simulink model "sampleModel20"  (R2021a)
settings: Solver=VariableStepAuto  StartTime=0.0  StopTime=10.0  RelTol=1e-3
undefined symbols (not defined in the file): DiscIntNeverNeededParam, magnitude, Newton, Raphson
libraries: simulink x274, pid_lib x17
(part 12 of 16)

== system sampleModel20/cfblk86/cfblk9/cfblk4/cfblk10 ==
  cfblk1 : Inport
  cfblk9 : Inport  Port=2
  cfblk10 : Inport  Port=3
  cfblk3 : Sqrt  Operator=rSqrt  AlgorithmType=Newton-Raphson  SaturateOnIntegerOverflow=on
  cfblk4 : UnaryMinus
  cfblk5 : Product  Inputs=*
  cfblk6 : PermuteDimensions
  cfblk7 : Sqrt  Operator=rSqrt  AlgorithmType=Newton-Raphson  SaturateOnIntegerOverflow=on
  cfblk8 : Sum  Inputs=+-
  cfblk2 : Outport
  wires:
  cfblk8/1 -> cfblk4/1
  cfblk6/1 -> cfblk2/1
  cfblk5/1 -> cfblk8/1
  cfblk1/1 -> cfblk7/1
  cfblk3/1 -> cfblk5/1
  cfblk10/1 -> cfblk8/2
  cfblk9/1 -> cfblk3/1
  cfblk4/1 -> cfblk6/1

== system sampleModel20/cfblk86/cfblk9/cfblk4/cfblk11 ==
  cfblk1 : Inport
  cfblk6 : Inport  Port=2
  cfblk7 : Inport  Port=3
  cfblk8 : Inport  Port=4
  cfblk9 : Inport  Port=5
  cfblk10 : Inport  Port=6
  cfblk3 : Squeeze
  cfblk4 : ComplexToMagnitudeAngle
  cfblk5 : Product  Inputs=*
  cfblk2 : Outport
  cfblk11 : Outport  Port=2
  wires:
  cfblk8/1 -> cfblk2/1
  cfblk6/1 -> cfblk4/1
  cfblk1/1 -> cfblk11/1
  cfblk4/1 -> cfblk5/1
  cfblk9/1 -> cfblk3/1

== system sampleModel20/cfblk86/cfblk9/cfblk4/cfblk12 ==
  cfblk1 : Inport
  cfblk9 : Inport  Port=2
  cfblk10 : Inport  Port=3
  cfblk11 : Inport  Port=4
  cfblk3 : Reshape
  cfblk4 : Math  Operator=mod  SaturateOnIntegerOverflow=on
  cfblk5 : DotProduct  InputSameDT=on  OutDataTypeStr=Inherit: Inherit via internal rule
  cfblk6 : Sum  Inputs=|++
  cfblk7 : Product  Inputs=**
  cfblk8 : PermuteDimensions
  cfblk2 : Outport
  wires:
  cfblk8/1 -> cfblk3/1
  cfblk11/1 -> cfblk7/1
  cfblk1/1 -> cfblk5/1
  cfblk3/1 -> cfblk7/2
  cfblk9/1 -> cfblk4/1
  cfblk10/1 -> cfblk4/2, cfblk5/2
  cfblk7/1 -> cfblk2/1
  cfblk6/1 -> cfblk8/1
  cfblk4/1 -> cfblk6/1
  cfblk5/1 -> cfblk6/2

== system sampleModel20/cfblk86/cfblk9/cfblk4/cfblk9 ==
  cfblk1 : Inport
  cfblk9 : Inport  Port=2
  cfblk10 : Inport  Port=3
  cfblk11 : Inport  Port=4
  cfblk13 : Delay  SampleTime=1
  cfblk3 : Squeeze
  cfblk4 : Sin  TimeSource=Use external signal  SampleTime=0
  cfblk5 : Sum  Inputs=+
  cfblk6 : simulink/Math Operations/MinMax Running Resettable  Function=min  vinit=0.0
  cfblk7 : Sum  Inputs=--
  cfblk8 : simulink/Math Operations/MinMax Running Resettable  Function=min  vinit=0.0
  cfblk2 : Outport
  cfblk12 : Outport  Port=2
  wires:
  cfblk8/1 -> cfblk4/1
  cfblk1/1 -> cfblk7/2
  cfblk10/1 -> cfblk2/1
  cfblk9/1 -> cfblk8/1
  cfblk7/1 -> cfblk3/1
  cfblk3/1 -> cfblk5/1, cfblk6/2
  cfblk11/1 -> cfblk8/2
  cfblk5/1 -> cfblk12/1
  cfblk4/1 -> cfblk6/1
  cfblk6/1 -> cfblk13/1
  cfblk13/1 -> cfblk7/1

== system sampleModel20/cfblk86/cfblk9/cfblk5/cfblk11 ==
  cfblk1 : Inport
  cfblk6 : Inport  Port=2
  cfblk7 : Inport  Port=3
  cfblk8 : Inport  Port=4
  cfblk9 : Inport  Port=5
  cfblk10 : Inport  Port=6
  cfblk11 : Inport  Port=7
  cfblk12 : Inport  Port=8
  cfblk3 : ComplexToMagnitudeAngle
  cfblk4 : Gain  Gain=[-542068454.447755]
  cfblk5 : Sqrt  SaturateOnIntegerOverflow=on
  cfblk2 : Outport
  cfblk13 : Outport  Port=2
  cfblk14 : Outport  Port=3
  cfblk15 : Outport  Port=4
  wires:
  cfblk3/1 -> cfblk5/1
  cfblk5/1 -> cfblk2/1
  cfblk7/1 -> cfblk4/1
  cfblk6/1 -> cfblk15/1
  cfblk10/1 -> cfblk3/1
  cfblk12/1 -> cfblk13/1
  cfblk3/2 -> cfblk14/1

== system sampleModel20/cfblk86/cfblk9/cfblk5/cfblk12 ==
  cfblk1 : Inport
  cfblk5 : Inport  Port=2
  cfblk6 : Inport  Port=3
  cfblk7 : Inport  Port=4
  cfblk3 : Assignment  DiagnosticForDimensions=Warning  IndexOptions=Index vector (dialog)  Indices=1  OutputSizes=1
  cfblk4 : Assignment  DiagnosticForDimensions=Warning  IndexOptions=Index vector (dialog)  Indices=1  OutputSizes=1
  cfblk2 : Outport
  cfblk8 : Outport  Port=2
  wires:
  cfblk6/1 -> cfblk4/1
  cfblk1/1 -> cfblk8/1
  cfblk7/1 -> cfblk3/1
  cfblk5/1 -> cfblk3/2
  cfblk4/1 -> cfblk2/1
  cfblk3/1 -> cfblk4/2

== system sampleModel20/cfblk86/cfblk9/cfblk6/cfblk6 ==
  cfblk1 : Inport
  cfblk8 : Inport  Port=2
  cfblk9 : Inport  Port=3
  cfblk10 : Inport  Port=4
  cfblk11 : Inport  Port=5
  cfblk3 : ComplexToRealImag
  cfblk4 : Polyval  Coefs=[ +2.081618890e-019, -1.441693666e-014, +4.719686976e-010, -8.536869453e-006, +1.621573104e-001, -8.087801117e+001 ]
  cfblk5 : ComplexToRealImag
  cfblk6 : Product  Inputs=**
  cfblk7 : Signum
  cfblk2 : Outport
  wires:
  cfblk11/1 -> cfblk6/1
  cfblk9/1 -> cfblk4/1
  cfblk10/1 -> cfblk7/1
  cfblk4/1 -> cfblk6/2
  cfblk3/1 -> cfblk5/1
  cfblk7/1 -> cfblk2/1
  cfblk1/1 -> cfblk3/1

== system sampleModel20/cfblk86/cfblk9/cfblk6/cfblk7 ==
  cfblk1 : Inport
  cfblk11 : Inport  Port=2
  cfblk12 : Inport  Port=3
  cfblk13 : Inport  Port=4
  cfblk14 : Inport  Port=5
  cfblk15 : Inport  Port=6
  cfblk10 : MinMax  Inputs=3
  cfblk3 : DiscreteFir  SampleTime=1
  cfblk4 : Assignment  DiagnosticForDimensions=Warning  IndexOptions=Index vector (dialog)  Indices=1  OutputSizes=1
  cfblk5 : Product  Inputs=**
  cfblk6 : Squeeze
  cfblk7 : Signum
  cfblk8 : ComplexToRealImag
  cfblk9 : Sqrt  Operator=rSqrt  AlgorithmType=Newton-Raphson  SaturateOnIntegerOverflow=on
  cfblk2 : Outport
  cfblk16 : Outport  Port=2
  wires:
  cfblk10/1 -> cfblk2/1
  cfblk13/1 -> cfblk6/1
  cfblk3/1 -> cfblk9/1
  cfblk12/1 -> cfblk7/1
  cfblk6/1 -> cfblk3/1
  cfblk4/1 -> cfblk16/1
  cfblk8/1 -> cfblk5/1
  cfblk7/1 -> cfblk8/1
  cfblk8/2 -> cfblk5/2
  cfblk9/1 -> cfblk10/1
  cfblk15/1 -> cfblk10/2
  cfblk1/1 -> cfblk10/3
  cfblk14/1 -> cfblk4/1
  cfblk5/1 -> cfblk4/2

== system sampleModel20/cfblk86/cfblk9/cfblk6/cfblk8 ==
  cfblk1 : Inport
  cfblk7 : Inport  Port=2
  cfblk8 : Inport  Port=3
  cfblk9 : Inport  Port=4
  cfblk10 : Inport  Port=5
  cfblk11 : Inport  Port=6
  cfblk3 : Sin  TimeSource=Use external signal  SampleTime=0
  cfblk4 : Product  Inputs=*
  cfblk5 : simulink/Math Operations/Slider Gain  gain=1  low=0  high=2
  cfblk6 : Reshape
  cfblk2 : Outport
  cfblk12 : Outport  Port=2
  cfblk13 : Outport  Port=3
  wires:
  cfblk1/1 -> cfblk6/1
  cfblk10/1 -> cfblk2/1
  cfblk8/1 -> cfblk12/1
  cfblk11/1 -> cfblk4/1
  cfblk7/1 -> cfblk3/1
  cfblk5/1 -> cfblk13/1
  cfblk3/1 -> cfblk5/1

== system sampleModel20/cfblk86/cfblk9/cfblk7/cfblk8 ==
  cfblk1 : Inport
  cfblk11 : Inport  Port=2
  cfblk12 : Inport  Port=3
  cfblk13 : Inport  Port=4
  cfblk14 : Inport  Port=5
  cfblk10 : ComplexToRealImag
  cfblk16 : Delay  SampleTime=1
  cfblk3 : Math  Operator=10^u  SaturateOnIntegerOverflow=on
  cfblk4 : Math  Operator=transpose  SaturateOnIntegerOverflow=on
  cfblk5 : Sqrt  Operator=rSqrt  AlgorithmType=Newton-Raphson  SaturateOnIntegerOverflow=on
  cfblk6 : Sqrt  Operator=rSqrt  AlgorithmType=Newton-Raphson  SaturateOnIntegerOverflow=on
  cfblk7 : Sum  Inputs=+
  cfblk8 : Rounding
  cfblk9 : Squeeze
  cfblk2 : Outport
  cfblk15 : Outport  Port=2
  wires:
  cfblk5/1 -> cfblk10/1
  cfblk7/1 -> cfblk9/1
  cfblk1/1 -> cfblk3/1
  cfblk14/1 -> cfblk5/1
  cfblk3/1 -> cfblk2/1
  cfblk4/1 -> cfblk6/1
  cfblk10/1 -> cfblk15/1
  cfblk11/1 -> cfblk8/1
  cfblk10/2 -> cfblk4/1
  cfblk9/1 -> cfblk16/1
  cfblk16/1 -> cfblk7/1

== system sampleModel20/cfblk86/cfblk9/cfblk8/cfblk4 ==
  cfblk1 : Inport
  cfblk6 : Inport  Port=2
  cfblk7 : Inport  Port=3
  cfblk8 : Inport  Port=4
  cfblk9 : Inport  Port=5
  cfblk10 : Inport  Port=6
  cfblk11 : Inport  Port=7
  cfblk3 : PermuteDimensions
  cfblk4 : ComplexToRealImag
  cfblk5 : Sin  TimeSource=Use external signal  SampleTime=0
  cfblk2 : Outport
  wires:
  cfblk4/1 -> cfblk5/1
  cfblk9/1 -> cfblk2/1
  cfblk4/2 -> cfblk3/1
  cfblk7/1 -> cfblk4/1

== system sampleModel20/cfblk86/cfblk9/cfblk8/cfblk5 ==
  cfblk1 : Inport
  cfblk9 : Inport  Port=2
  cfblk10 : Inport  Port=3
  cfblk11 : Inport  Port=4
  cfblk12 : Inport  Port=5
  cfblk13 : Inport  Port=6
  cfblk16 : Delay  SampleTime=1
  cfblk3 : Reshape
  cfblk4 : Math  Operator=transpose  SaturateOnIntegerOverflow=on
  cfblk5 : Sqrt  SaturateOnIntegerOverflow=on
  cfblk6 : PermuteDimensions
  cfblk7 : UnaryMinus
  cfblk8 : Trigonometry
  cfblk2 : Outport
  cfblk14 : Outport  Port=2
  cfblk15 : Outport  Port=3
  wires:
  cfblk10/1 -> cfblk7/1
  cfblk3/1 -> cfblk8/1
  cfblk7/1 -> cfblk6/1
  cfblk12/1 -> cfblk2/1
  cfblk1/1 -> cfblk5/1
  cfblk6/1 -> cfblk4/1
  cfblk4/1 -> cfblk15/1
  cfblk11/1 -> cfblk14/1
  cfblk8/1 -> cfblk16/1
  cfblk16/1 -> cfblk3/1

== system sampleModel20/cfblk86/cfblk9/cfblk8/cfblk6 ==
  cfblk1 : Inport
  cfblk7 : Inport  Port=2
  cfblk8 : Inport  Port=3
  cfblk9 : Inport  Port=4
  cfblk3 : Product  Inputs=*
  cfblk4 : ComplexToRealImag
  cfblk5 : Squeeze
  cfblk6 : Sum  Inputs=|++
  cfblk2 : Outport
  wires:
  cfblk3/1 -> cfblk4/1
  cfblk1/1 -> cfblk6/1
  cfblk8/1 -> cfblk3/1
  cfblk9/1 -> cfblk2/1
  cfblk7/1 -> cfblk5/1
  cfblk4/1 -> cfblk6/2

== system sampleModel20/cfblk86/cfblk9/cfblk8/cfblk7 ==
  cfblk1 : Inport
  cfblk11 : Inport  Port=2
  cfblk12 : Inport  Port=3
  cfblk13 : Inport  Port=4
  cfblk14 : Inport  Port=5
  cfblk15 : Inport  Port=6
  cfblk10 : Squeeze
  cfblk18 : Delay  SampleTime=1
  cfblk19 : Delay  SampleTime=1
  cfblk3 : ComplexToMagnitudeAngle
  cfblk4 : MinMax  Function=max  Inputs=2
  cfblk5 : Squeeze
  cfblk6 : Sum
  cfblk7 : Sum  Inputs=|++
  cfblk8 : PermuteDimensions
  cfblk9 : ComplexToRealImag
  cfblk2 : Outport
  cfblk16 : Outport  Port=2
  cfblk17 : Outport  Port=3
  wires:
  cfblk14/1 -> cfblk8/1
  cfblk12/1 -> cfblk10/1
  cfblk1/1 -> cfblk2/1
  cfblk7/1 -> cfblk5/1
  cfblk15/1 -> cfblk6/1
  cfblk11/1 -> cfblk7/1
  cfblk3/1 -> cfblk6/2
  cfblk6/1 -> cfblk9/1
  cfblk8/1 -> cfblk4/1
  cfblk4/1 -> cfblk7/2
  cfblk9/2 -> cfblk16/1
  cfblk10/1 -> cfblk17/1
  cfblk9/1 -> cfblk18/1
  cfblk18/1 -> cfblk3/1
  cfblk5/1 -> cfblk19/1
  cfblk19/1 -> cfblk4/2

== system sampleModel20/cfblk86/cfblk9/cfblk9/cfblk10 ==
  cfblk1 : Inport
  cfblk10 : Inport  Port=2
  cfblk11 : Inport  Port=3
  cfblk16 : Delay  SampleTime=1
  cfblk17 : Delay  SampleTime=1
  cfblk3 : Squeeze
  cfblk4 : Sum  Inputs=+-
  cfblk5 : Trigonometry
  cfblk6 : Product  Inputs=*
  cfblk7 : Rounding
  cfblk8 : Gain  Gain=[414263899.014972]
  cfblk9 : Sin  TimeSource=Use external signal  SampleTime=0
  cfblk2 : Outport
  cfblk12 : Outport  Port=2
  cfblk13 : Outport  Port=3
  cfblk14 : Outport  Port=4
  cfblk15 : Outport  Port=5
  wires:
  cfblk6/1 -> cfblk12/1, cfblk16/1
  cfblk11/1 -> cfblk14/1
  cfblk9/1 -> cfblk2/1
  cfblk10/1 -> cfblk9/1
  cfblk4/1 -> cfblk6/1
  cfblk5/1 -> cfblk15/1
  cfblk8/1 -> cfblk5/1, cfblk4/1
  cfblk1/1 -> cfblk8/1
  cfblk3/1 -> cfblk7/1, cfblk13/1
  cfblk16/1 -> cfblk4/2
  cfblk7/1 -> cfblk17/1
  cfblk17/1 -> cfblk3/1

== system sampleModel20/cfblk86/cfblk9/cfblk9/cfblk6 ==
  cfblk1 : Inport
  cfblk11 : Inport  Port=2
  cfblk12 : Inport  Port=3
  cfblk13 : Inport  Port=4
  cfblk10 : Rounding
  cfblk16 : Delay  SampleTime=1
  cfblk3 : Sum  Inputs=|++
  cfblk4 : Bias  Bias=[573429226.430379]
  cfblk5 : Sum  Inputs=+
  cfblk6 : Abs
  cfblk7 : Trigonometry
  cfblk8 : MinMax  Inputs=3
  cfblk9 : ComplexToMagnitudeAngle
  cfblk2 : Outport
  cfblk14 : Outport  Port=2
  cfblk15 : Outport  Port=3
  wires:
  cfblk5/1 -> cfblk10/1
  cfblk9/1 -> cfblk7/1
  cfblk9/2 -> cfblk2/1
  cfblk11/1 -> cfblk14/1
  cfblk13/1 -> cfblk9/1
  cfblk7/1 -> cfblk8/1
  cfblk6/1 -> cfblk5/1
  cfblk3/1 -> cfblk4/1
  cfblk10/1 -> cfblk15/1, cfblk8/3
  cfblk12/1 -> cfblk8/2
  cfblk8/1 -> cfblk3/2
  cfblk1/1 -> cfblk6/1
  cfblk4/1 -> cfblk16/1
  cfblk16/1 -> cfblk3/1

== system sampleModel20/cfblk86/cfblk9/cfblk9/cfblk7 ==
  cfblk1 : Inport
  cfblk7 : Inport  Port=2
  cfblk8 : Inport  Port=3
  cfblk9 : Inport  Port=4
  cfblk10 : Inport  Port=5
  cfblk11 : Inport  Port=6
  cfblk12 : Inport  Port=7
  cfblk3 : Polyval  Coefs=[ +2.081618890e-019, -1.441693666e-014, +4.719686976e-010, -8.536869453e-006, +1.621573104e-001, -8.087801117e+001 ]
  cfblk4 : simulink/Math Operations/MinMax Running Resettable  Function=min  vinit=0.0
  cfblk5 : DotProduct  InputSameDT=on  OutDataTypeStr=Inherit: Inherit via internal rule
  cfblk6 : Sin  TimeSource=Use external signal  SampleTime=0
  cfblk2 : Outport
  cfblk13 : Outport  Port=2
  wires:
  cfblk10/1 -> cfblk3/1
  cfblk4/1 -> cfblk13/1
  cfblk12/1 -> cfblk5/1
  cfblk6/1 -> cfblk2/1
  cfblk3/1 -> cfblk4/1
  cfblk11/1 -> cfblk6/1
  cfblk7/1 -> cfblk4/2
  cfblk8/1 -> cfblk5/2

== system sampleModel20/cfblk86/cfblk9/cfblk9/cfblk8 ==
  cfblk1 : Inport
  cfblk9 : Inport  Port=2
  cfblk10 : Inport  Port=3
  cfblk12 : Delay  SampleTime=1
  cfblk3 : Sum  Inputs=|++
  cfblk4 : Sin  TimeSource=Use external signal  SampleTime=0
  cfblk5 : PermuteDimensions
  cfblk6 : PermuteDimensions
  cfblk7 : Bias  Bias=[458708821.734373]
  cfblk8 : UnaryMinus
  cfblk2 : Outport
  cfblk11 : Outport  Port=2
  wires:
  cfblk8/1 -> cfblk7/1
  cfblk4/1 -> cfblk5/1
  cfblk7/1 -> cfblk6/1
  cfblk9/1 -> cfblk11/1
  cfblk10/1 -> cfblk8/1
  cfblk3/1 -> cfblk2/1
  cfblk6/1 -> cfblk3/1
  cfblk1/1 -> cfblk3/2
  cfblk5/1 -> cfblk12/1
  cfblk12/1 -> cfblk4/1

== system sampleModel20/cfblk86/cfblk9/cfblk9/cfblk9 ==
  cfblk1 : Inport
  cfblk7 : Inport  Port=2
  cfblk8 : Inport  Port=3
  cfblk3 : simulink/Math Operations/MinMax Running Resettable  Function=min  vinit=0.0
  cfblk4 : Reshape
  cfblk5 : Math  SaturateOnIntegerOverflow=on
  cfblk6 : Sum  Inputs=+-
  cfblk9 : Delay  SampleTime=1
  cfblk2 : Outport
  wires:
  cfblk6/1 -> cfblk3/1
  cfblk7/1 -> cfblk5/1
  cfblk1/1 -> cfblk6/1
  cfblk5/1 -> cfblk2/1
  cfblk3/1 -> cfblk4/1
  cfblk8/1 -> cfblk6/2
  cfblk4/1 -> cfblk9/1
  cfblk9/1 -> cfblk3/2

== system sampleModel20/cfblk87/cfblk5/cfblk10/cfblk6 ==
  cfblk1 : Inport
  cfblk10 : Inport  Port=2
  cfblk11 : Inport  Port=3
  cfblk12 : Inport  Port=4
  cfblk13 : Inport  Port=5
  cfblk14 : Inport  Port=6
  cfblk3 : DotProduct  InputSameDT=on  OutDataTypeStr=Inherit: Inherit via internal rule
  cfblk4 : Sum  Inputs=+-
  cfblk5 : Sqrt  Operator=rSqrt  AlgorithmType=Newton-Raphson  SaturateOnIntegerOverflow=on
  cfblk6 : Sum  Inputs=+-
  cfblk7 : Gain  Gain=[158003740.430733]
  cfblk8 : Sum  Inputs=--
  cfblk9 : Constant  Value=[-369906265.637833]  SampleTime=1
  cfblk2 : Outport
  cfblk15 : Outport  Port=2
  wires:
  cfblk8/1 -> cfblk15/1
  cfblk14/1 -> cfblk5/1
  cfblk7/1 -> cfblk6/1
  cfblk10/1 -> cfblk7/1
  cfblk9/1 -> cfblk4/1
  cfblk12/1 -> cfblk3/1
  cfblk3/1 -> cfblk6/2
  cfblk5/1 -> cfblk3/2
  cfblk1/1 -> cfblk4/2
  cfblk6/1 -> cfblk2/1
  cfblk4/1 -> cfblk8/1
  cfblk11/1 -> cfblk8/2

== system sampleModel20/cfblk87/cfblk5/cfblk11/cfblk10 ==
  cfblk1 : Inport
  cfblk11 : Inport  Port=2
  cfblk12 : Inport  Port=3
  cfblk13 : Inport  Port=4
  cfblk14 : Inport  Port=5
  cfblk10 : MinMax  Function=max
  cfblk3 : Bias  Bias=[224777352.991120]
  cfblk4 : Squeeze
  cfblk5 : Math  Operator=log10  SaturateOnIntegerOverflow=on
  cfblk6 : Polyval  Coefs=[ +2.081618890e-019, -1.441693666e-014, +4.719686976e-010, -8.536869453e-006, +1.621573104e-001, -8.087801117e+001 ]
  cfblk7 : ComplexToMagnitudeAngle
  cfblk8 : Gain  Gain=[-96724518.527223]
  cfblk9 : ComplexToRealImag
  cfblk2 : Outport
  wires:
  cfblk4/1 -> cfblk2/1
  cfblk6/1 -> cfblk3/1
  cfblk9/1 -> cfblk4/1
  cfblk7/1 -> cfblk10/1
  cfblk8/1 -> cfblk6/1
  cfblk12/1 -> cfblk5/1
  cfblk3/1 -> cfblk9/1
  cfblk14/1 -> cfblk7/1
  cfblk11/1 -> cfblk8/1

== system sampleModel20/cfblk87/cfblk5/cfblk11/cfblk8 ==
  cfblk1 : Inport
  cfblk7 : Inport  Port=2
  cfblk8 : Inport  Port=3
  cfblk9 : Inport  Port=4
  cfblk10 : Inport  Port=5
  cfblk11 : Inport  Port=6
  cfblk12 : Inport  Port=7
  cfblk13 : Inport  Port=8
  cfblk3 : Rounding
  cfblk4 : MinMax  Inputs=3
  cfblk5 : Reshape
  cfblk6 : UnaryMinus
  cfblk2 : Outport
  cfblk14 : Outport  Port=2
  cfblk15 : Outport  Port=3
  cfblk16 : Outport  Port=4
  wires:
  cfblk8/1 -> cfblk14/1
  cfblk6/1 -> cfblk2/1
  cfblk1/1 -> cfblk3/1
  cfblk12/1 -> cfblk5/1
  cfblk3/1 -> cfblk6/1
  cfblk9/1 -> cfblk16/1
  cfblk13/1 -> cfblk4/1
  cfblk10/1 -> cfblk4/2
  cfblk5/1 -> cfblk4/3
  cfblk7/1 -> cfblk15/1

== system sampleModel20/cfblk87/cfblk5/cfblk11/cfblk9 ==
  cfblk1 : Inport
  cfblk11 : Inport  Port=2
  cfblk12 : Inport  Port=3
  cfblk13 : Inport  Port=4
  cfblk14 : Inport  Port=5
  cfblk10 : Sqrt  SaturateOnIntegerOverflow=on
  cfblk3 : DiscreteFir  SampleTime=1
  cfblk4 : Trigonometry
  cfblk5 : Polyval  Coefs=[ +2.081618890e-019, -1.441693666e-014, +4.719686976e-010, -8.536869453e-006, +1.621573104e-001, -8.087801117e+001 ]
  cfblk6 : Gain  Gain=[-825576826.966571]
  cfblk7 : Signum
  cfblk8 : Sum  Inputs=|++
  cfblk9 : simulink/Math Operations/Slider Gain  gain=1  low=0  high=2
  cfblk2 : Outport
  cfblk15 : Outport  Port=2
  wires:
  cfblk4/1 -> cfblk8/1
  cfblk11/1 -> cfblk9/1
  cfblk7/1 -> cfblk10/1
  cfblk8/1 -> cfblk15/1
  cfblk10/1 -> cfblk2/1
  cfblk5/1 -> cfblk8/2
  cfblk14/1 -> cfblk3/1
  cfblk13/1 -> cfblk7/1
  cfblk1/1 -> cfblk4/1
  cfblk3/1 -> cfblk6/1
  cfblk9/1 -> cfblk5/1

== system sampleModel20/cfblk87/cfblk5/cfblk7/cfblk7 ==
  cfblk1 : Inport
  cfblk4 : Inport  Port=2
  cfblk5 : Inport  Port=3
  cfblk6 : Inport  Port=4
  cfblk7 : Inport  Port=5
  cfblk8 : Inport  Port=6
  cfblk9 : Inport  Port=7
  cfblk3 : ComplexToMagnitudeAngle
  cfblk2 : Outport
  wires:
  cfblk9/1 -> cfblk2/1
  cfblk7/1 -> cfblk3/1

== system sampleModel20/cfblk87/cfblk5/cfblk8/cfblk10 ==
  cfblk1 : Inport
  cfblk9 : Inport  Port=2
  cfblk10 : Delay  SampleTime=1
  cfblk3 : Abs
  cfblk4 : Signum
  cfblk5 : Sum  Inputs=+
  cfblk6 : ComplexToMagnitudeAngle
  cfblk7 : Product  Inputs=**
  cfblk8 : Reshape
  cfblk2 : Outport
  wires:
  cfblk9/1 -> cfblk2/1
  cfblk4/1 -> cfblk3/1
  cfblk3/1 -> cfblk6/1
  cfblk8/1 -> cfblk5/1
  cfblk7/1 -> cfblk4/1
  cfblk1/1 -> cfblk7/1
  cfblk6/1 -> cfblk8/1
  cfblk6/2 -> cfblk10/1
  cfblk10/1 -> cfblk7/2

== system sampleModel20/cfblk87/cfblk5/cfblk8/cfblk7 ==
  cfblk1 : Inport
  cfblk10 : Inport  Port=2
  cfblk11 : Inport  Port=3
  cfblk12 : Inport  Port=4
  cfblk13 : Inport  Port=5
  cfblk14 : Delay  SampleTime=1
  cfblk3 : simulink/Math Operations/MinMax Running Resettable  Function=min  vinit=0.0
  cfblk4 : Assignment  DiagnosticForDimensions=Warning  IndexOptions=Index vector (dialog)  Indices=1  OutputSizes=1
  cfblk5 : Sum  Inputs=+
  cfblk6 : Reshape
  cfblk7 : Trigonometry
  cfblk8 : Sqrt  Operator=rSqrt  AlgorithmType=Newton-Raphson  SaturateOnIntegerOverflow=on
  cfblk9 : Polyval  Coefs=[ +2.081618890e-019, -1.441693666e-014, +4.719686976e-010, -8.536869453e-006, +1.621573104e-001, -8.087801117e+001 ]
  cfblk2 : Outport
  wires:
  cfblk3/1 -> cfblk5/1
  cfblk11/1 -> cfblk7/1
  cfblk4/1 -> cfblk3/2
  cfblk7/1 -> cfblk6/1
  cfblk13/1 -> cfblk4/1
  cfblk8/1 -> cfblk4/2
  cfblk10/1 -> cfblk2/1
  cfblk12/1 -> cfblk9/1
  cfblk6/1 -> cfblk8/1
  cfblk5/1 -> cfblk14/1
  cfblk14/1 -> cfblk3/1

== system sampleModel20/cfblk87/cfblk5/cfblk8/cfblk8 ==
  cfblk1 : Inport
  cfblk7 : Inport  Port=2
  cfblk8 : Inport  Port=3
  cfblk9 : Inport  Port=4
  cfblk3 : ComplexToMagnitudeAngle
  cfblk4 : Signum
  cfblk5 : Abs
  cfblk6 : ComplexToRealImag
  cfblk2 : Outport
  cfblk10 : Outport  Port=2
  cfblk11 : Outport  Port=3
  wires:
  cfblk4/1 -> cfblk3/1
  cfblk8/1 -> cfblk10/1
  cfblk6/1 -> cfblk11/1
  cfblk9/1 -> cfblk6/1
  cfblk5/1 -> cfblk4/1
  cfblk7/1 -> cfblk2/1
  cfblk1/1 -> cfblk5/1

== system sampleModel20/cfblk87/cfblk5/cfblk8/cfblk9 ==
  cfblk1 : Inport
  cfblk7 : Inport  Port=2
  cfblk8 : Inport  Port=3
  cfblk9 : Inport  Port=4
  cfblk13 : Delay  SampleTime=1
  cfblk3 : Trigonometry
  cfblk4 : Signum
  cfblk5 : Product  Inputs=*
  cfblk6 : Sum  Inputs=+-
  cfblk2 : Outport
  cfblk10 : Outport  Port=2
  cfblk11 : Outport  Port=3
  cfblk12 : Outport  Port=4
  wires:
  cfblk5/1 -> cfblk3/1
  cfblk9/1 -> cfblk11/1
  cfblk1/1 -> cfblk6/1
  cfblk8/1 -> cfblk2/1
  cfblk7/1 -> cfblk4/1
  cfblk6/1 -> cfblk10/1, cfblk5/1
  cfblk4/1 -> cfblk12/1
  cfblk3/1 -> cfblk13/1
  cfblk13/1 -> cfblk6/2

== system sampleModel20/cfblk87/cfblk5/cfblk9/cfblk5 ==
  cfblk1 : Inport
  cfblk7 : Inport  Port=2
  cfblk8 : Inport  Port=3
  cfblk9 : Inport  Port=4
  cfblk10 : Inport  Port=5
  cfblk11 : Inport  Port=6
  cfblk12 : Inport  Port=7
  cfblk13 : Inport  Port=8
  cfblk14 : Inport  Port=9
  cfblk15 : Inport  Port=10
  cfblk3 : Squeeze
  cfblk4 : simulink/Math Operations/Slider Gain  gain=1  low=0  high=2
  cfblk5 : simulink/Math Operations/MinMax Running Resettable  Function=min  vinit=0.0
  cfblk6 : Sqrt  SaturateOnIntegerOverflow=on
  cfblk2 : Outport
  cfblk16 : Outport  Port=2
  cfblk17 : Outport  Port=3
  wires:
  cfblk5/1 -> cfblk3/1
  cfblk10/1 -> cfblk16/1
  cfblk8/1 -> cfblk6/1
  cfblk3/1 -> cfblk17/1
  cfblk11/1 -> cfblk4/1
  cfblk9/1 -> cfblk5/1
  cfblk13/1 -> cfblk5/2
  cfblk1/1 -> cfblk2/1

== system sampleModel20/cfblk87/cfblk5/cfblk9/cfblk6 ==
  cfblk1 : Inport
  cfblk7 : Inport  Port=2
  cfblk8 : Inport  Port=3
  cfblk9 : Inport  Port=4
  cfblk3 : simulink/Math Operations/Slider Gain  gain=1  low=0  high=2
  cfblk4 : Sum  Inputs=--
  cfblk5 : Gain  Gain=[915664602.907245]
  cfblk6 : Sum  Inputs=+-
  cfblk2 : Outport
  wires:
  cfblk1/1 -> cfblk4/1
  cfblk7/1 -> cfblk2/1
  cfblk6/1 -> cfblk4/2
  cfblk8/1 -> cfblk3/1
  cfblk3/1 -> cfblk5/1
  cfblk5/1 -> cfblk6/1
  cfblk9/1 -> cfblk6/2

== system sampleModel20/cfblk87/cfblk6/cfblk10/cfblk4 ==
  cfblk1 : Inport
  cfblk8 : Inport  Port=2
  cfblk9 : Inport  Port=3
  cfblk10 : Inport  Port=4
  cfblk13 : Delay  SampleTime=1
  cfblk3 : ComplexToRealImag
  cfblk4 : Sqrt  SaturateOnIntegerOverflow=on
  cfblk5 : PermuteDimensions
  cfblk6 : Assignment  DiagnosticForDimensions=Warning  IndexOptions=Index vector (dialog)  Indices=1  OutputSizes=1
  cfblk7 : UnaryMinus
  cfblk2 : Outport
  cfblk11 : Outport  Port=2
  cfblk12 : Outport  Port=3
  wires:
  cfblk10/1 -> cfblk12/1
  cfblk4/1 -> cfblk2/1
  cfblk3/1 -> cfblk11/1
  cfblk6/1 -> cfblk7/1
  cfblk9/1 -> cfblk6/1
  cfblk1/1 -> cfblk4/1
  cfblk5/1 -> cfblk6/2
  cfblk8/1 -> cfblk3/1
  cfblk7/1 -> cfblk13/1
  cfblk13/1 -> cfblk5/1

== system sampleModel20/cfblk87/cfblk6/cfblk10/cfblk5 ==
  cfblk1 : Inport
  cfblk7 : Inport  Port=2
  cfblk8 : Inport  Port=3
  cfblk9 : Inport  Port=4
  cfblk10 : Inport  Port=5
  cfblk3 : MinMax
  cfblk4 : Sum  Inputs=|++
  cfblk5 : Squeeze
  cfblk6 : Abs
  cfblk2 : Outport
  cfblk11 : Outport  Port=2
  cfblk12 : Outport  Port=3
  wires:
  cfblk7/1 -> cfblk2/1
  cfblk8/1 -> cfblk12/1
  cfblk9/1 -> cfblk3/1
  cfblk3/1 -> cfblk5/1
  cfblk6/1 -> cfblk11/1
  cfblk5/1 -> cfblk6/1
  cfblk10/1 -> cfblk4/1
  cfblk1/1 -> cfblk4/2

== system sampleModel20/cfblk87/cfblk6/cfblk10/cfblk6 ==
  cfblk1 : Inport
  cfblk5 : Inport  Port=2
  cfblk6 : Inport  Port=3
  cfblk3 : Assignment  DiagnosticForDimensions=Warning  IndexOptions=Index vector (dialog)  Indices=1  OutputSizes=1
  cfblk4 : DotProduct  InputSameDT=on  OutDataTypeStr=Inherit: Inherit via internal rule
  cfblk8 : Delay  SampleTime=1
  cfblk2 : Outport
  cfblk7 : Outport  Port=2
  wires:
  cfblk1/1 -> cfblk2/1
  cfblk3/1 -> cfblk7/1, cfblk4/2
  cfblk6/1 -> cfblk3/2
  cfblk5/1 -> cfblk4/1
  cfblk4/1 -> cfblk8/1
  cfblk8/1 -> cfblk3/1

== system sampleModel20/cfblk87/cfblk6/cfblk10/cfblk7 ==
  cfblk1 : Inport
  cfblk6 : Inport  Port=2
  cfblk7 : Inport  Port=3
  cfblk8 : Inport  Port=4
  cfblk9 : Inport  Port=5
  cfblk10 : Inport  Port=6
  cfblk3 : ComplexToMagnitudeAngle
  cfblk4 : MinMax  Function=max
  cfblk5 : Abs
  cfblk2 : Outport
  wires:
  cfblk8/1 -> cfblk2/1
  cfblk6/1 -> cfblk5/1
  cfblk9/1 -> cfblk4/1
  cfblk1/1 -> cfblk3/1

== system sampleModel20/cfblk87/cfblk6/cfblk11/cfblk4 ==
  cfblk1 : Inport
  cfblk6 : Inport  Port=2
  cfblk7 : Inport  Port=3
  cfblk8 : Inport  Port=4
  cfblk3 : Sum  Inputs=+
  cfblk4 : Sum  Inputs=|++
  cfblk5 : MinMax  Inputs=3
  cfblk2 : Outport
  cfblk9 : Outport  Port=2
  cfblk10 : Outport  Port=3
  cfblk11 : Outport  Port=4
  wires:
  cfblk5/1 -> cfblk4/1
  cfblk1/1 -> cfblk3/1
  cfblk6/1 -> cfblk4/2, cfblk5/2, cfblk5/3
  cfblk8/1 -> cfblk2/1
  cfblk7/1 -> cfblk5/1
  cfblk3/1 -> cfblk11/1
  cfblk4/1 -> cfblk10/1, cfblk9/1

== system sampleModel20/cfblk87/cfblk6/cfblk11/cfblk5 ==
  cfblk1 : Inport
  cfblk9 : Inport  Port=2
  cfblk10 : Inport  Port=3
  cfblk11 : Inport  Port=4
  cfblk12 : Inport  Port=5
  cfblk13 : Inport  Port=6
  cfblk14 : Inport  Port=7
  cfblk3 : Sin  TimeSource=Use external signal  SampleTime=0
  cfblk4 : Trigonometry
  cfblk5 : Reshape
  cfblk6 : DotProduct  InputSameDT=on  OutDataTypeStr=Inherit: Inherit via internal rule
  cfblk7 : MinMax  Function=max  Inputs=3
  cfblk8 : Sum  Inputs=|++
  cfblk2 : Outport
  cfblk15 : Outport  Port=2
  cfblk16 : Outport  Port=3
  wires:
  cfblk12/1 -> cfblk3/1
  cfblk10/1 -> cfblk4/1
  cfblk9/1 -> cfblk2/1
  cfblk3/1 -> cfblk5/1
  cfblk14/1 -> cfblk8/1
  cfblk8/1 -> cfblk15/1
  cfblk1/1 -> cfblk7/1
  cfblk5/1 -> cfblk7/2
  cfblk13/1 -> cfblk7/3
  cfblk4/1 -> cfblk8/2
  cfblk11/1 -> cfblk6/1
  cfblk7/1 -> cfblk6/2
  cfblk6/1 -> cfblk16/1

== system sampleModel20/cfblk87/cfblk6/cfblk12/cfblk10 ==
  cfblk1 : Inport
  cfblk4 : Inport  Port=2
  cfblk5 : Inport  Port=3
  cfblk6 : Inport  Port=4
  cfblk7 : Inport  Port=5
  cfblk8 : Inport  Port=6
  cfblk9 : Inport  Port=7
  cfblk3 : Squeeze
  cfblk2 : Outport
  cfblk10 : Outport  Port=2
  cfblk11 : Outport  Port=3
  wires:
  cfblk9/1 -> cfblk11/1
  cfblk3/1 -> cfblk10/1
  cfblk1/1 -> cfblk3/1
  cfblk4/1 -> cfblk2/1

== system sampleModel20/cfblk87/cfblk6/cfblk12/cfblk11 ==
  cfblk1 : Inport
  cfblk8 : Inport  Port=2
  cfblk9 : Inport  Port=3
  cfblk10 : Inport  Port=4
  cfblk11 : Inport  Port=5
  cfblk12 : Inport  Port=6
  cfblk13 : Inport  Port=7
  cfblk14 : Inport  Port=8
  cfblk15 : Inport  Port=9
  cfblk3 : Rounding
  cfblk4 : simulink/Math Operations/Slider Gain  gain=1  low=0  high=2
  cfblk5 : Product  Inputs=**
  cfblk6 : Sum  Inputs=|++
  cfblk7 : Sum  Inputs=+
  cfblk2 : Outport
  cfblk16 : Outport  Port=2
  cfblk17 : Outport  Port=3
  wires:
  cfblk13/1 -> cfblk5/1
  cfblk12/1 -> cfblk17/1
  cfblk6/1 -> cfblk16/1
  cfblk14/1 -> cfblk3/1
  cfblk7/1 -> cfblk5/2
  cfblk5/1 -> cfblk4/1
  cfblk9/1 -> cfblk7/1
  cfblk1/1 -> cfblk6/1
  cfblk3/1 -> cfblk2/1
  cfblk10/1 -> cfblk6/2

== system sampleModel20/cfblk87/cfblk6/cfblk12/cfblk7 ==
  cfblk1 : Inport
  cfblk9 : Inport  Port=2
  cfblk10 : Inport  Port=3
  cfblk11 : Inport  Port=4
  cfblk12 : Inport  Port=5
  cfblk13 : Inport  Port=6
  cfblk14 : Inport  Port=7
  cfblk15 : Inport  Port=8
  cfblk3 : Product  Inputs=*
  cfblk4 : simulink/Math Operations/MinMax Running Resettable  Function=min  vinit=0.0
  cfblk5 : Trigonometry
  cfblk6 : Squeeze
  cfblk7 : DotProduct  InputSameDT=on  OutDataTypeStr=Inherit: Inherit via internal rule
  cfblk8 : Signum
  cfblk2 : Outport
  wires:
  cfblk11/1 -> cfblk3/1
  cfblk8/1 -> cfblk5/1
  cfblk13/1 -> cfblk6/1
  cfblk1/1 -> cfblk4/1
  cfblk6/1 -> cfblk8/1
  cfblk5/1 -> cfblk7/1
  cfblk4/1 -> cfblk2/1
  cfblk9/1 -> cfblk4/2
  cfblk12/1 -> cfblk7/2

== system sampleModel20/cfblk87/cfblk6/cfblk12/cfblk8 ==
  cfblk1 : Inport
  cfblk7 : Inport  Port=2
  cfblk8 : Inport  Port=3
  cfblk3 : ComplexToMagnitudeAngle
  cfblk4 : Squeeze
  cfblk5 : Product  Inputs=*
  cfblk6 : ComplexToMagnitudeAngle
  cfblk2 : Outport
  wires:
  cfblk6/1 -> cfblk3/1
  cfblk5/1 -> cfblk6/1
  cfblk7/1 -> cfblk4/1
  cfblk4/1 -> cfblk2/1
  cfblk1/1 -> cfblk5/1

== system sampleModel20/cfblk87/cfblk6/cfblk12/cfblk9 ==
  cfblk1 : Inport
  cfblk9 : Inport  Port=2
  cfblk10 : Inport  Port=3
  cfblk11 : Inport  Port=4
  cfblk12 : Inport  Port=5
  cfblk13 : Inport  Port=6
  cfblk16 : Delay  SampleTime=1
  cfblk3 : Sqrt  SaturateOnIntegerOverflow=on
  cfblk4 : Product  Inputs=**
  cfblk5 : ComplexToMagnitudeAngle
  cfblk6 : Product  Inputs=**
  cfblk7 : Squeeze
  cfblk8 : Math  Operator=hermitian  SaturateOnIntegerOverflow=on
  cfblk2 : Outport
  cfblk14 : Outport  Port=2
  cfblk15 : Outport  Port=3
  wires:
  cfblk8/1 -> cfblk2/1
  cfblk5/1 -> cfblk4/1
  cfblk10/1 -> cfblk8/1
  cfblk13/1 -> cfblk7/1
  cfblk6/1 -> cfblk15/1
  cfblk9/1 -> cfblk5/1
  cfblk1/1 -> cfblk14/1
  cfblk11/1 -> cfblk6/1
  cfblk3/1 -> cfblk4/2
  cfblk7/1 -> cfblk6/2
  cfblk4/1 -> cfblk16/1
  cfblk16/1 -> cfblk3/1

== system sampleModel20/cfblk87/cfblk7/cfblk10/cfblk10 ==
  cfblk1 : Inport
  cfblk5 : Inport  Port=2
  cfblk6 : Inport  Port=3
  cfblk7 : Inport  Port=4
  cfblk3 : Sqrt  Operator=rSqrt  AlgorithmType=Newton-Raphson  SaturateOnIntegerOverflow=on
  cfblk4 : Rounding
  cfblk2 : Outport
  wires:
  cfblk7/1 -> cfblk4/1
  cfblk4/1 -> cfblk3/1
  cfblk3/1 -> cfblk2/1

== system sampleModel20/cfblk87/cfblk7/cfblk10/cfblk11 ==
  cfblk1 : Inport
  cfblk7 : Inport  Port=2
  cfblk8 : Inport  Port=3
  cfblk3 : Reshape
  cfblk4 : Product  Inputs=*
  cfblk5 : Sum
  cfblk6 : Sum  Inputs=+-
  cfblk9 : Delay  SampleTime=1
  cfblk2 : Outport
  wires:
  cfblk6/1 -> cfblk2/1
  cfblk8/1 -> cfblk4/1
  cfblk1/1 -> cfblk6/1
  cfblk7/1 -> cfblk5/1
  cfblk4/1 -> cfblk6/2
  cfblk3/1 -> cfblk5/2
  cfblk5/1 -> cfblk9/1
  cfblk9/1 -> cfblk3/1

== system sampleModel20/cfblk87/cfblk7/cfblk10/cfblk12 ==
  cfblk1 : Inport
  cfblk8 : Inport  Port=2
  cfblk9 : Inport  Port=3
  cfblk10 : Inport  Port=4
  cfblk11 : Inport  Port=5
  cfblk12 : Inport  Port=6
  cfblk13 : Inport  Port=7
  cfblk14 : Inport  Port=8
  cfblk3 : DiscreteTransferFcn  SampleTime=1
  cfblk4 : Rounding
  cfblk5 : Math  Operator=log10  SaturateOnIntegerOverflow=on
  cfblk6 : Polyval  Coefs=[ +2.081618890e-019, -1.441693666e-014, +4.719686976e-010, -8.536869453e-006, +1.621573104e-001, -8.087801117e+001 ]
  cfblk7 : Abs
  cfblk2 : Outport
  cfblk15 : Outport  Port=2
  cfblk16 : Outport  Port=3
  wires:
  cfblk9/1 -> cfblk7/1
  cfblk10/1 -> cfblk5/1
  cfblk3/1 -> cfblk2/1
  cfblk1/1 -> cfblk4/1
  cfblk8/1 -> cfblk3/1
  cfblk13/1 -> cfblk6/1
  cfblk14/1 -> cfblk16/1
  cfblk5/1 -> cfblk15/1

== system sampleModel20/cfblk87/cfblk7/cfblk11/cfblk10 ==
  cfblk1 : Inport
  cfblk7 : Inport  Port=2
  cfblk8 : Inport  Port=3
  cfblk3 : Delay  DelayLengthSource=Input port  SampleTime=1
      settings: InputPortMap=u0,p1
  cfblk4 : Sqrt  Operator=rSqrt  AlgorithmType=Newton-Raphson  SaturateOnIntegerOverflow=on
  cfblk5 : Product  Inputs=**
  cfblk6 : Signum
  cfblk2 : Outport
  wires:
  cfblk7/1 -> cfblk3/1
  cfblk3/1 -> cfblk4/1
  cfblk4/1 -> cfblk5/1
  cfblk6/1 -> cfblk3/2
  cfblk8/1 -> cfblk6/1
  cfblk1/1 -> cfblk5/2
  cfblk5/1 -> cfblk2/1

== system sampleModel20/cfblk87/cfblk7/cfblk11/cfblk11 ==
  cfblk1 : Inport
  cfblk6 : Inport  Port=2
  cfblk7 : Inport  Port=3
  cfblk8 : Inport  Port=4
  cfblk9 : Inport  Port=5
  cfblk3 : Bias  Bias=[379857874.439988]
  cfblk4 : UnaryMinus
  cfblk5 : Rounding
  cfblk2 : Outport
  cfblk10 : Outport  Port=2
  cfblk11 : Outport  Port=3
  cfblk12 : Outport  Port=4
  wires:
  cfblk6/1 -> cfblk2/1
  cfblk5/1 -> cfblk3/1
  cfblk8/1 -> cfblk5/1
  cfblk1/1 -> cfblk10/1
  cfblk3/1 -> cfblk4/1
  cfblk7/1 -> cfblk11/1
  cfblk4/1 -> cfblk12/1

== system sampleModel20/cfblk87/cfblk7/cfblk11/cfblk6 ==
  cfblk1 : Inport
  cfblk11 : Inport  Port=2
  cfblk12 : Inport  Port=3
  cfblk13 : Inport  Port=4
  cfblk14 : Inport  Port=5
  cfblk15 : Inport  Port=6
  cfblk16 : Inport  Port=7
  cfblk10 : MinMax  Inputs=2
  cfblk3 : DiscreteStateSpace
  cfblk4 : Product
  cfblk5 : Squeeze
  cfblk6 : ComplexToRealImag
  cfblk7 : Abs
  cfblk8 : UnaryMinus
  cfblk9 : simulink/Math Operations/Slider Gain  gain=1  low=0  high=2
  cfblk2 : Outport
  wires:
  cfblk13/1 -> cfblk4/1
  cfblk15/1 -> cfblk2/1
  cfblk8/1 -> cfblk3/1
  cfblk14/1 -> cfblk4/2
  cfblk7/1 -> cfblk8/1
  cfblk3/1 -> cfblk6/1
  cfblk16/1 -> cfblk9/1
  cfblk11/1 -> cfblk7/1
  cfblk10/1 -> cfblk5/1
  cfblk9/1 -> cfblk10/1
  cfblk1/1 -> cfblk10/2

== system sampleModel20/cfblk87/cfblk7/cfblk11/cfblk7 ==
  cfblk1 : Inport
  cfblk8 : Inport  Port=2
  cfblk9 : Inport  Port=3
  cfblk10 : Inport  Port=4
  cfblk11 : Inport  Port=5
  cfblk12 : Inport  Port=6
  cfblk13 : Inport  Port=7
  cfblk14 : Inport  Port=8
  cfblk3 : ComplexToMagnitudeAngle
  cfblk4 : Squeeze
  cfblk5 : UnaryMinus
  cfblk6 : Math  Operator=hermitian  SaturateOnIntegerOverflow=on
  cfblk7 : Product  Inputs=**
  cfblk2 : Outport
  cfblk15 : Outport  Port=2
  cfblk16 : Outport  Port=3
  cfblk17 : Outport  Port=4
  wires:
  cfblk5/1 -> cfblk4/1
  cfblk10/1 -> cfblk5/1
  cfblk13/1 -> cfblk2/1
  cfblk6/1 -> cfblk16/1
  cfblk1/1 -> cfblk17/1
  cfblk4/1 -> cfblk7/1
  cfblk12/1 -> cfblk3/1
  cfblk14/1 -> cfblk6/1
  cfblk9/1 -> cfblk7/2
  cfblk7/1 -> cfblk15/1

== system sampleModel20/cfblk87/cfblk7/cfblk11/cfblk8 ==
  cfblk1 : Inport
  cfblk7 : Inport  Port=2
  cfblk8 : Inport  Port=3
  cfblk9 : Inport  Port=4
  cfblk3 : Sin  TimeSource=Use external signal  SampleTime=0
  cfblk4 : Rounding
  cfblk5 : Product  Inputs=**
  cfblk6 : Rounding
  cfblk2 : Outport
  wires:
  cfblk6/1 -> cfblk5/1
  cfblk1/1 -> cfblk4/1
  cfblk7/1 -> cfblk6/1
  cfblk8/1 -> cfblk3/1
  cfblk5/1 -> cfblk2/1
  cfblk4/1 -> cfblk5/2

== system sampleModel20/cfblk87/cfblk7/cfblk11/cfblk9 ==
  cfblk1 : Inport
  cfblk8 : Inport  Port=2
  cfblk9 : Inport  Port=3
  cfblk10 : Inport  Port=4
  cfblk11 : Inport  Port=5
  cfblk3 : Reshape
  cfblk4 : Sin  TimeSource=Use external signal  SampleTime=0
  cfblk5 : Sqrt  Operator=rSqrt  AlgorithmType=Newton-Raphson  SaturateOnIntegerOverflow=on
  cfblk6 : Polyval  Coefs=[ +2.081618890e-019, -1.441693666e-014, +4.719686976e-010, -8.536869453e-006, +1.621573104e-001, -8.087801117e+001 ]
  cfblk7 : Abs
  cfblk2 : Outport
  wires:
  cfblk11/1 -> cfblk7/1
  cfblk1/1 -> cfblk5/1
  cfblk4/1 -> cfblk6/1
  cfblk7/1 -> cfblk4/1
  cfblk5/1 -> cfblk2/1
  cfblk9/1 -> cfblk3/1

== system sampleModel20/cfblk87/cfblk7/cfblk12/cfblk10 ==
  cfblk1 : Inport
  cfblk14 : Inport  Port=2
  cfblk15 : Inport  Port=3
  cfblk10 : Squeeze
  cfblk11 : Product  Inputs=*
  cfblk12 : ComplexToMagnitudeAngle
  cfblk13 : Polyval  Coefs=[ +2.081618890e-019, -1.441693666e-014, +4.719686976e-010, -8.536869453e-006, +1.621573104e-001, -8.087801117e+001 ]
  cfblk18 : Delay  SampleTime=1
  cfblk19 : Delay  SampleTime=1
  cfblk3 : simulink/Discrete/Transfer Fcn First Order  PoleZ=0.95  ICPrevOutput=0.0  DoSatur=off
  cfblk4 : Delay  ShowEnablePort=on  SampleTime=1
      settings: InputPortMap=u0,e6
  cfblk5 : ComplexToRealImag
  cfblk6 : DotProduct  InputSameDT=on  OutDataTypeStr=Inherit: Inherit via internal rule
  cfblk7 : Trigonometry
  cfblk8 : Sin  TimeSource=Use external signal  SampleTime=0
  cfblk9 : Polyval  Coefs=[ +2.081618890e-019, -1.441693666e-014, +4.719686976e-010, -8.536869453e-006, +1.621573104e-001, -8.087801117e+001 ]
  cfblk2 : Outport
  cfblk16 : Outport  Port=2
  cfblk17 : Outport  Port=3
  wires:
  cfblk4/1 -> cfblk12/1
  cfblk10/1 -> cfblk5/1
  cfblk7/1 -> cfblk9/1
  cfblk15/1 -> cfblk10/1
  cfblk3/1 -> cfblk7/1
  cfblk1/1 -> cfblk17/1
  cfblk11/1 -> cfblk16/1
  cfblk14/1 -> cfblk4/2
  cfblk5/1 -> cfblk8/1
  cfblk8/1 -> cfblk11/1
  cfblk12/1 -> cfblk6/1
  cfblk5/2 -> cfblk2/1
  cfblk12/2 -> cfblk6/2
  cfblk6/1 -> cfblk13/1
  cfblk9/1 -> cfblk18/1
  cfblk18/1 -> cfblk3/1
  cfblk13/1 -> cfblk19/1
  cfblk19/1 -> cfblk4/1

== system sampleModel20/cfblk87/cfblk7/cfblk12/cfblk11 ==
  cfblk1 : Inport
  cfblk6 : Inport  Port=2
  cfblk7 : Inport  Port=3
  cfblk3 : pid_lib/PID Controller  Controller=PID  Form=Parallel  TimeDomain=Discrete-time  UseExternalTs=off  SampleTime=1  IntegratorMethod=Forward Euler  FilterMethod=Forward Euler  ControllerParametersSource=internal  P=1  I=1  D=0  UseFilter=on  N=100  TunerSelectOption=Transfer Function Based (PID Tuner App)  InitialConditionSource=internal  InitialConditionForIntegrator=0  InitialConditionForFilter=0  DifferentiatorICPrevScaledInput=0  ExternalReset=none  TrackingMode=off  Kt=1  LimitOutput=off  SatLimitsSource=internal  UpperSaturationLimit=inf  LowerSaturationLimit=-inf  LinearizeAsGain=off  AntiWindupMode=none  Kb=1  POutMin=[]  POutMax=[]  IOutMin=[]  IOutMax=[]  DOutMin=[]  DOutMax=[]  NOutMin=[]  NOutMax=[]  SumOutMin=[]  SumOutMax=[]  SaturationOutMin=[]  SaturationOutMax=[]  PParamMin=[]  PParamMax=[]  IParamMin=[]  IParamMax=[]  DParamMin=[]  DParamMax=[]  NParamMin=[]  NParamMax=[]  KbParamMin=[]  KbParamMax=[]  KtParamMin=[]  KtParamMax=[]  KbOutMin=[]  KbOutMax=[]  KtOutMin=[]  KtOutMax=[]  IntegratorOutMin=[]  IntegratorOutMax=[]  FilterOutMin=[]  FilterOutMax=[]  SumI1OutMin=[]  SumI1OutMax=[]  SumI2OutMin=[]  SumI2OutMax=[]  SumI3OutMin=[]  SumI3OutMax=[]  SumI4OutMin=[]  SumI4OutMax=[]  SumDOutMin=[]  SumDOutMax=[]  DifferentiatorOutMin=[]  DifferentiatorOutMax=[]  FilterDiffOutCoefMin=[]  FilterDiffOutCoefMax=[]  ReciprocalOutMin=[]  ReciprocalOutMax=[]  SumDenOutMin=[]  SumDenOutMax=[]  SumNumOutMin=[]  SumNumOutMax=[]  DivideOutMin=[]  DivideOutMax=[]  UdiffTsProdOutMin=[]  UdiffTsProdOutMax=[]  NTsProdOutMin=[]  NTsProdOutMax=[]  UintegralTsProdOutMin=[]  UintegralTsProdOutMax=[]  UngainTsProdOutMin=[]  UngainTsProdOutMax=[]  IntegratorContinuousStateAttributes=''  IntegratorStateMustResolveToSignalObject=off  IntegratorRTWStateStorageClass=Auto  FilterContinuousStateAttributes=''  FilterStateMustResolveToSignalObject=off  FilterRTWStateStorageClass=Auto  ParallelPVariant=InternalParameters  IdealPVariant=Disabled  IVariant=InternalParameters  DVariant=InternalParameters  IntegratorVariant=Discrete  SatVariant=Disabled  AWVariant=Passthrough  PCopyVariant=Disabled  TRVariant=Disabled  FdbkBlocksVariant=Forward  IdealPFdbkVariant=Disabled  SatFdbkVariant=Disabled  DerivativeFilterVariant=ForwardEulerFilter  NVariant=InternalParameters  NCopyVariant=Disabled  FilterICVariant=InternalICsFilter  IntegratorICVariant=InternalICs  ExternalResetVariant=Disabled  TRSumVariant=Passthrough  SumFdbkVariant=Disabled  SumVariant=Sum_PID  TsampFilterVariant=InternalTs  TsampNgainVariant=Passthrough  TsampIntegralVariant=Passthrough  ExternalSaturationOutDataTypeStr=Inherit: Same as second input
  cfblk4 : Reshape
  cfblk5 : ComplexToRealImag
  cfblk2 : Outport
  wires:
  cfblk5/1 -> cfblk3/1
  cfblk5/2 -> cfblk2/1
  cfblk1/1 -> cfblk5/1
  cfblk3/1 -> cfblk4/1

== system sampleModel20/cfblk87/cfblk7/cfblk12/cfblk12 ==
  cfblk1 : Inport
  cfblk14 : Inport  Port=2
  cfblk15 : Inport  Port=3
  cfblk16 : Inport  Port=4
  cfblk10 : Product  Inputs=*
  cfblk11 : MinMax
  cfblk12 : Polyval  Coefs=[ +2.081618890e-019, -1.441693666e-014, +4.719686976e-010, -8.536869453e-006, +1.621573104e-001, -8.087801117e+001 ]
  cfblk13 : MinMax  Inputs=3
  cfblk18 : Delay  SampleTime=1
  cfblk19 : Delay  SampleTime=1
  cfblk3 : Sum  Inputs=+-
  cfblk4 : MinMax  Function=max  Inputs=2
  cfblk5 : Trigonometry
  cfblk6 : DotProduct  InputSameDT=on  OutDataTypeStr=Inherit: Inherit via internal rule
  cfblk7 : ComplexToMagnitudeAngle
  cfblk8 : Product
  cfblk9 : Product  Inputs=**
  cfblk2 : Outport
  cfblk17 : Outport  Port=2
  wires:
  cfblk9/1 -> cfblk17/1
  cfblk3/1 -> cfblk7/1
  cfblk11/1 -> cfblk13/1
  cfblk7/1 -> cfblk2/1
  cfblk15/1 -> cfblk5/1
  cfblk5/1 -> cfblk12/1
  cfblk8/1 -> cfblk6/1
  cfblk10/1 -> cfblk11/1, cfblk19/1
  cfblk7/2 -> cfblk10/1
  cfblk16/1 -> cfblk9/1
  cfblk1/1 -> cfblk3/1, cfblk8/2, cfblk4/2
  cfblk12/1 -> cfblk9/2
  cfblk13/1 -> cfblk8/1
  cfblk14/1 -> cfblk6/2, cfblk13/3
  cfblk6/1 -> cfblk4/1
  cfblk4/1 -> cfblk18/1
  cfblk18/1 -> cfblk13/2
  cfblk19/1 -> cfblk3/2

== system sampleModel20/cfblk87/cfblk7/cfblk12/cfblk9 ==
  cfblk1 : Inport
  cfblk5 : Inport  Port=2
  cfblk6 : Inport  Port=3
  cfblk7 : Inport  Port=4
  cfblk3 : Abs
  cfblk4 : Polyval  Coefs=[ +2.081618890e-019, -1.441693666e-014, +4.719686976e-010, -8.536869453e-006, +1.621573104e-001, -8.087801117e+001 ]
  cfblk2 : Outport
  cfblk8 : Outport  Port=2
  wires:
  cfblk6/1 -> cfblk4/1
  cfblk4/1 -> cfblk3/1
  cfblk5/1 -> cfblk2/1
  cfblk1/1 -> cfblk8/1

== system sampleModel20/cfblk87/cfblk7/cfblk9/cfblk10 ==
  cfblk1 : Inport
  cfblk6 : Inport  Port=2
  cfblk7 : Inport  Port=3
  cfblk8 : Inport  Port=4
  cfblk9 : Inport  Port=5
  cfblk3 : Reshape
  cfblk4 : Product
  cfblk5 : simulink/Math Operations/MinMax Running Resettable  Function=min  vinit=0.0
  cfblk2 : Outport
  wires:
  cfblk5/1 -> cfblk2/1
  cfblk4/1 -> cfblk5/1
  cfblk3/1 -> cfblk5/2
  cfblk6/1 -> cfblk3/1
  cfblk8/1 -> cfblk4/1
  cfblk7/1 -> cfblk4/2

== system sampleModel20/cfblk87/cfblk7/cfblk9/cfblk11 ==
  cfblk1 : Inport
  cfblk4 : Inport  Port=2
  cfblk5 : Inport  Port=3
  cfblk6 : Inport  Port=4
  cfblk3 : Product
  cfblk2 : Outport
  cfblk7 : Outport  Port=2
  wires:
  cfblk6/1 -> cfblk7/1
  cfblk4/1 -> cfblk3/1
  cfblk1/1 -> cfblk2/1
  cfblk5/1 -> cfblk3/2

== system sampleModel20/cfblk87/cfblk7/cfblk9/cfblk7 ==
  cfblk1 : Inport
  cfblk4 : Inport  Port=2
  cfblk5 : Inport  Port=3
  cfblk6 : Inport  Port=4
  cfblk7 : Inport  Port=5
  cfblk3 : Assignment  DiagnosticForDimensions=Warning  IndexOptions=Index vector (dialog)  Indices=1  OutputSizes=1
  cfblk2 : Outport
  wires:
  cfblk7/1 -> cfblk3/1
  cfblk4/1 -> cfblk3/2
  cfblk5/1 -> cfblk2/1

== system sampleModel20/cfblk87/cfblk7/cfblk9/cfblk8 ==
  cfblk1 : Inport
  cfblk7 : Inport  Port=2
  cfblk8 : Inport  Port=3
  cfblk9 : Inport  Port=4
  cfblk3 : simulink/Math Operations/Slider Gain  gain=1  low=0  high=2
  cfblk4 : Bias  Bias=[398847297.986755]
  cfblk5 : ComplexToRealImag
  cfblk6 : Abs
  cfblk2 : Outport
  cfblk10 : Outport  Port=2
  wires:
  cfblk8/1 -> cfblk2/1
  cfblk3/1 -> cfblk10/1
  cfblk1/1 -> cfblk3/1
  cfblk7/1 -> cfblk6/1
  cfblk6/1 -> cfblk5/1
  cfblk5/1 -> cfblk4/1

== system sampleModel20/cfblk87/cfblk7/cfblk9/cfblk9 ==
  cfblk1 : Inport
  cfblk3 : Math  Operator=transpose  SaturateOnIntegerOverflow=on
  cfblk4 : Bias  Bias=[179400792.820333]
  cfblk5 : Sum  Inputs=+
  cfblk6 : Gain  Gain=[-494254179.392719]
  cfblk2 : Outport
  cfblk7 : Outport  Port=2
  wires:
  cfblk6/1 -> cfblk5/1
  cfblk4/1 -> cfblk2/1
  cfblk3/1 -> cfblk6/1, cfblk4/1
  cfblk5/1 -> cfblk7/1
  cfblk1/1 -> cfblk3/1

== system sampleModel20/cfblk87/cfblk8/cfblk6/cfblk12 ==
  cfblk1 : Inport
  cfblk6 : Inport  Port=2
  cfblk3 : UnaryMinus
  cfblk4 : ComplexToMagnitudeAngle
  cfblk5 : Signum
  cfblk2 : Outport
  cfblk7 : Outport  Port=2
  wires:
  cfblk1/1 -> cfblk2/1
  cfblk5/1 -> cfblk7/1
  cfblk6/1 -> cfblk3/1
  cfblk3/1 -> cfblk5/1, cfblk4/1

== system sampleModel20/cfblk87/cfblk8/cfblk6/cfblk13 ==
  cfblk1 : Inport
  cfblk8 : Inport  Port=2
  cfblk9 : Inport  Port=3
  cfblk10 : Inport  Port=4
  cfblk12 : Delay  SampleTime=1
  cfblk3 : Reshape
  cfblk4 : Sum  Inputs=+-
  cfblk5 : Polyval  Coefs=[ +2.081618890e-019, -1.441693666e-014, +4.719686976e-010, -8.536869453e-006, +1.621573104e-001, -8.087801117e+001 ]
  cfblk6 : Math  Operator=rem  SaturateOnIntegerOverflow=on
  cfblk7 : Sum  Inputs=+-
  cfblk2 : Outport
  cfblk11 : Outport  Port=2
  wires:
  cfblk6/1 -> cfblk5/1, cfblk7/2
  cfblk3/1 -> cfblk4/1
  cfblk4/1 -> cfblk6/1
  cfblk8/1 -> cfblk3/1
  cfblk10/1 -> cfblk6/2
  cfblk1/1 -> cfblk11/1
  cfblk9/1 -> cfblk7/1
  cfblk5/1 -> cfblk2/1
  cfblk7/1 -> cfblk12/1
  cfblk12/1 -> cfblk4/2

== system sampleModel20/cfblk87/cfblk8/cfblk7/cfblk3 ==
  cfblk1 : Inport
  cfblk10 : Inport  Port=2
  cfblk11 : Inport  Port=3
  cfblk12 : Inport  Port=4
  cfblk13 : Inport  Port=5
  cfblk14 : Inport  Port=6
  cfblk18 : Delay  SampleTime=1
  cfblk19 : Delay  SampleTime=1
  cfblk3 : Product  Inputs=*
  cfblk4 : Sum  Inputs=+-
  cfblk5 : Sum  Inputs=+-
  cfblk6 : Abs
  cfblk7 : Gain  Gain=[-604533193.703964]
  cfblk8 : PermuteDimensions
  cfblk9 : Sum  Inputs=+-
  cfblk2 : Outport
  cfblk15 : Outport  Port=2
  cfblk16 : Outport  Port=3
  cfblk17 : Outport  Port=4
  wires:
  cfblk4/1 -> cfblk7/1
  cfblk1/1 -> cfblk16/1
  cfblk14/1 -> cfblk2/1
  cfblk7/1 -> cfblk15/1, cfblk19/1
  cfblk3/1 -> cfblk9/1
  cfblk11/1 -> cfblk5/1
  cfblk10/1 -> cfblk17/1
  cfblk8/1 -> cfblk5/2
  cfblk6/1 -> cfblk3/1
  cfblk9/1 -> cfblk8/1
  cfblk13/1 -> cfblk6/1
  cfblk12/1 -> cfblk4/1
  cfblk5/1 -> cfblk18/1
  cfblk18/1 -> cfblk9/2
  cfblk19/1 -> cfblk4/2

== system sampleModel20/cfblk87/cfblk9/cfblk5/cfblk10 ==
  cfblk1 : Inport
  cfblk9 : Inport  Port=2
  cfblk10 : Inport  Port=3
  cfblk11 : Inport  Port=4
  cfblk3 : Reshape
  cfblk4 : simulink/Math Operations/Slider Gain  gain=1  low=0  high=2
  cfblk5 : Polyval  Coefs=[ +2.081618890e-019, -1.441693666e-014, +4.719686976e-010, -8.536869453e-006, +1.621573104e-001, -8.087801117e+001 ]
  cfblk6 : Polyval  Coefs=[ +2.081618890e-019, -1.441693666e-014, +4.719686976e-010, -8.536869453e-006, +1.621573104e-001, -8.087801117e+001 ]
  cfblk7 : UnaryMinus
  cfblk8 : Reshape
  cfblk2 : Outport
  cfblk12 : Outport  Port=2
  wires:
  cfblk9/1 -> cfblk6/1
  cfblk7/1 -> cfblk8/1
  cfblk8/1 -> cfblk12/1
  cfblk4/1 -> cfblk5/1
  cfblk5/1 -> cfblk2/1
  cfblk11/1 -> cfblk7/1
  cfblk6/1 -> cfblk4/1
  cfblk10/1 -> cfblk3/1

== system sampleModel20/cfblk87/cfblk9/cfblk5/cfblk11 ==
  cfblk1 : Inport
  cfblk11 : Inport  Port=2
  cfblk12 : Inport  Port=3
  cfblk13 : Inport  Port=4
  cfblk10 : MinMax  Inputs=2
  cfblk16 : Delay  SampleTime=1
  cfblk3 : Assignment  DiagnosticForDimensions=Warning  IndexOptions=Index vector (dialog)  Indices=1  OutputSizes=1
  cfblk4 : Sqrt  Operator=rSqrt  AlgorithmType=Newton-Raphson  SaturateOnIntegerOverflow=on
  cfblk5 : Polyval  Coefs=[ +2.081618890e-019, -1.441693666e-014, +4.719686976e-010, -8.536869453e-006, +1.621573104e-001, -8.087801117e+001 ]
  cfblk6 : UnaryMinus
  cfblk7 : Abs
  cfblk8 : Trigonometry
  cfblk9 : Sum  Inputs=+-
  cfblk2 : Outport
  cfblk14 : Outport  Port=2
  cfblk15 : Outport  Port=3
  wires:
  cfblk3/1 -> cfblk6/1
  cfblk11/1 -> cfblk7/1
  cfblk13/1 -> cfblk14/1
  cfblk9/1 -> cfblk3/1
  cfblk1/1 -> cfblk5/1
  cfblk5/1 -> cfblk10/1, cfblk8/1
  cfblk8/1 -> cfblk2/1
  cfblk10/1 -> cfblk9/1
  cfblk4/1 -> cfblk9/2
  cfblk7/1 -> cfblk4/1, cfblk15/1
  cfblk12/1 -> cfblk10/2
  cfblk6/1 -> cfblk16/1
  cfblk16/1 -> cfblk3/2

== system sampleModel20/cfblk87/cfblk9/cfblk5/cfblk12 ==
  cfblk1 : Inport
  cfblk11 : Inport  Port=2
  cfblk10 : Reshape
  cfblk13 : Delay  SampleTime=1
  cfblk3 : ComplexToMagnitudeAngle
  cfblk4 : Sum  Inputs=+
  cfblk5 : Signum
  cfblk6 : Squeeze
  cfblk7 : DotProduct  InputSameDT=on  OutDataTypeStr=Inherit: Inherit via internal rule
  cfblk8 : Rounding
  cfblk9 : Gain  Gain=[-296987850.316911]
  cfblk2 : Outport
  cfblk12 : Outport  Port=2
  wires:
  cfblk11/1 -> cfblk8/1
  cfblk5/1 -> cfblk7/1
  cfblk1/1 -> cfblk5/1
  cfblk8/1 -> cfblk6/1
  cfblk3/1 -> cfblk2/1
  cfblk9/1 -> cfblk10/1
  cfblk6/1 -> cfblk12/1
  cfblk3/2 -> cfblk4/1
  cfblk10/1 -> cfblk3/1
  cfblk7/1 -> cfblk9/1
  cfblk4/1 -> cfblk13/1
  cfblk13/1 -> cfblk7/2

== system sampleModel20/cfblk87/cfblk9/cfblk5/cfblk13 ==
  cfblk1 : Inport
  cfblk9 : Inport  Port=2
  cfblk10 : Inport  Port=3
  cfblk12 : Delay  SampleTime=1
  cfblk3 : Squeeze
  cfblk4 : DotProduct  InputSameDT=on  OutDataTypeStr=Inherit: Inherit via internal rule
  cfblk5 : Sum  Inputs=|++
  cfblk6 : PermuteDimensions
  cfblk7 : Sqrt  Operator=rSqrt  AlgorithmType=Newton-Raphson  SaturateOnIntegerOverflow=on
  cfblk8 : Squeeze
  cfblk2 : Outport
  cfblk11 : Outport  Port=2
  wires:
  cfblk9/1 -> cfblk2/1
  cfblk1/1 -> cfblk7/1
  cfblk3/1 -> cfblk4/1
  cfblk7/1 -> cfblk6/1, cfblk5/2
  cfblk6/1 -> cfblk11/1
  cfblk10/1 -> cfblk4/2
  cfblk8/1 -> cfblk3/1
  cfblk5/1 -> cfblk8/1
  cfblk4/1 -> cfblk12/1
  cfblk12/1 -> cfblk5/1

== system sampleModel20/cfblk87/cfblk9/cfblk5/cfblk7 ==
  cfblk1 : Inport
  cfblk8 : Inport  Port=2
  cfblk9 : Inport  Port=3
  cfblk10 : Inport  Port=4
  cfblk11 : Inport  Port=5
  cfblk12 : Inport  Port=6
  cfblk13 : Inport  Port=7
  cfblk3 : Squeeze
  cfblk4 : Abs
  cfblk5 : DotProduct  InputSameDT=on  OutDataTypeStr=Inherit: Inherit via internal rule
  cfblk6 : Reshape
  cfblk7 : Gain  Gain=[802694218.765924]
  cfblk2 : Outport
  wires:
  cfblk10/1 -> cfblk6/1
  cfblk11/1 -> cfblk5/1
  cfblk12/1 -> cfblk4/1
  cfblk5/1 -> cfblk2/1
  cfblk4/1 -> cfblk7/1
  cfblk9/1 -> cfblk3/1
  cfblk8/1 -> cfblk5/2

== system sampleModel20/cfblk87/cfblk9/cfblk5/cfblk8 ==
  cfblk1 : Inport
  cfblk9 : Inport  Port=2
  cfblk10 : Inport  Port=3
  cfblk11 : Inport  Port=4
  cfblk12 : Inport  Port=5
  cfblk13 : Inport  Port=6
  cfblk14 : Inport  Port=7
  cfblk3 : UnaryMinus
  cfblk4 : Sum  Inputs=+
  cfblk5 : Gain  Gain=[-867749796.416216]
  cfblk6 : Trigonometry
  cfblk7 : Squeeze
  cfblk8 : Assignment  DiagnosticForDimensions=Warning  IndexOptions=Index vector (dialog)  Indices=1  OutputSizes=1
  cfblk2 : Outport
  cfblk15 : Outport  Port=2
  wires:
  cfblk8/1 -> cfblk15/1
  cfblk12/1 -> cfblk5/1
  cfblk4/1 -> cfblk7/1
  cfblk7/1 -> cfblk2/1
  cfblk10/1 -> cfblk8/1
  cfblk1/1 -> cfblk8/2
  cfblk5/1 -> cfblk3/1
  cfblk6/1 -> cfblk4/1
  cfblk3/1 -> cfblk6/1

== system sampleModel20/cfblk87/cfblk9/cfblk5/cfblk9 ==
  cfblk1 : Inport
  cfblk8 : Inport  Port=2
  cfblk9 : Inport  Port=3
  cfblk10 : Inport  Port=4
  cfblk3 : simulink/Math Operations/MinMax Running Resettable  Function=min  vinit=0.0
  cfblk4 : Trigonometry
  cfblk5 : Polyval  Coefs=[ +2.081618890e-019, -1.441693666e-014, +4.719686976e-010, -8.536869453e-006, +1.621573104e-001, -8.087801117e+001 ]
  cfblk6 : simulink/Math Operations/MinMax Running Resettable  Function=min  vinit=0.0
  cfblk7 : Sin  TimeSource=Use external signal  SampleTime=0
  cfblk2 : Outport
  cfblk11 : Outport  Port=2
  cfblk12 : Outport  Port=3
  cfblk13 : Outport  Port=4
  cfblk14 : Outport  Port=5
  cfblk15 : Outport  Port=6
  wires:
  cfblk6/1 -> cfblk14/1
  cfblk3/1 -> cfblk7/1
  cfblk7/1 -> cfblk5/1
  cfblk1/1 -> cfblk11/1
  cfblk5/1 -> cfblk2/1, cfblk6/2
  cfblk8/1 -> cfblk4/1, cfblk6/1
  cfblk4/1 -> cfblk15/1, cfblk12/1
  cfblk10/1 -> cfblk13/1, cfblk3/2
  cfblk9/1 -> cfblk3/1
